simulink model "md11fl"  (Simulink 7.5)
settings: Solver=ode45  StartTime=0.0  StopTime=20  RelTol=1e-3
values from neighbouring files (symbols this model uses):
  alpha1f = 2.5e-7    (= 2.5e-07)    [gsnew2011.m]    (also in md11fla2011.m)
  alpha2f = 0.025    [gsnew2011.m]    (also in md11fla2011.m)
  alpha3f = 1    [gsnew2011.m]    (also in md11fla2011.m)
  ap = [Xu Xw 0 -g;Zu Zw Zq 0;Mu Mw Mq 0;0 0 1 0]    [gsnew2011.m]    (also in md11fla2011.m = [Xu Xw 0 -g 0;Zu Zw Zq 0 0;Mu Mw Mq 0 0;0 0 1 0 0;0 -1/U0  0)
  bp = [XL XT XR;ZL ZT ZR;ML MT MR;0 0 0]    [gsnew2011.m]    (also in md11fla2011.m = [XL XT XR;ZL ZT ZR;ML MT MR;0 0 0; 0 0 0])
  Cpf = [1 0 0 0 0 0 0 0;0 1 0 0 0 0 0 0;0 0 0 U0 0 0 0 0;0 0 0 0 1 0 0 0]    [md11fla2011.m]
  h_cr = 15    [gsnew2011.m]    (also in md11fla2011.m = 15000)
  Kfl1 = Kfl(:,1:8)    [md11fla2011.m]
  Kfl2 = Kgs(:,9:10)    [md11fla2011.m]
  ncon = 3    [gsnew2011.m]    (also in md11fla2011.m)
  np = 4    [gsnew2011.m]    (also in md11fla2011.m = 5)
  pthrot = 0.6    [gsnew2011.m]    (also in md11fla2011.m = 1)
  T2 = 200    [md11fla2011.m]
  tou = 1    [md11fla2011.m]
  u_ref = 0    [gsnew2011.m]    (also in md11fla2011.m = 165)
settings Model: Creator=ranjan  LastModifiedBy=knightofaccess
settings OptimizationCC: InitFltsAndDblsToZero=on
settings DebuggingCC: StrictBusMsg=Warning

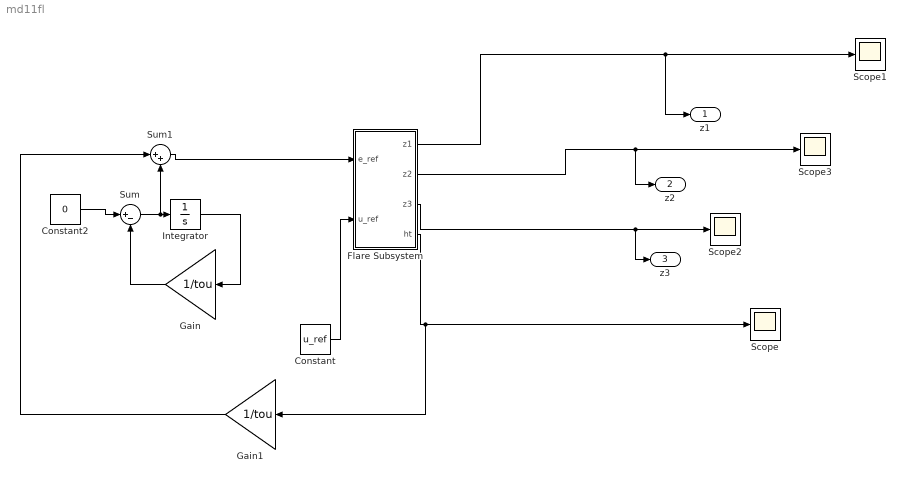
== system md11fl ==
  Constant : Constant  Value=u_ref  OutDataType=sfix(16)  OutScaling=2^0
  Constant2 : Constant  Value=0  OutDataType=sfix(16)  OutScaling=2^0
  Flare Subsystem : Subsystem
  Gain : Gain  Gain=1/tou  ParameterDataType=sfix(16)  ParameterScaling=2^0  OutDataType=sfix(16)  OutScaling=2^0
  Gain1 : Gain  Gain=1/tou  ParameterDataType=sfix(16)  ParameterScaling=2^0  OutDataType=sfix(16)  OutScaling=2^0
  Integrator : Integrator  InitialCondition=h_cr
  Scope{,1..3} (4 alike) : Scope
      Scope settings: YMin=-75600  YMax=-74950
      Scope2 settings: SaveName=ScopeData2
      Scope3 settings: SaveName=ScopeData3
  Sum : Sum  Inputs=|+-  OutDataType=sfix(16)  OutScaling=2^0
  Sum1 : Sum  Inputs=|++  OutDataType=sfix(16)  OutScaling=2^0
  z1 : Outport  OutDataType=sfix(16)  OutScaling=2^0
  z2 : Outport  Port=2  OutDataType=sfix(16)  OutScaling=2^0
  z3 : Outport  Port=3  OutDataType=sfix(16)  OutScaling=2^0
  wires:
  Constant/1 -> Flare Subsystem/2(u_ref)
  Flare Subsystem/1(z1) -> z1/1, Scope1/1
  Flare Subsystem/2(z2) -> z2/1, Scope3/1
  Flare Subsystem/3(z3) -> z3/1, Scope2/1
  Sum/1 -> Integrator/1, Sum1/2
  Constant2/1 -> Sum/1
  Integrator/1 -> Gain/1
  Gain/1 -> Sum/2
  Sum1/1 -> Flare Subsystem/1(e_ref)
  Flare Subsystem/4(ht) -> Scope/1, Gain1/1
  Gain1/1 -> Sum1/1

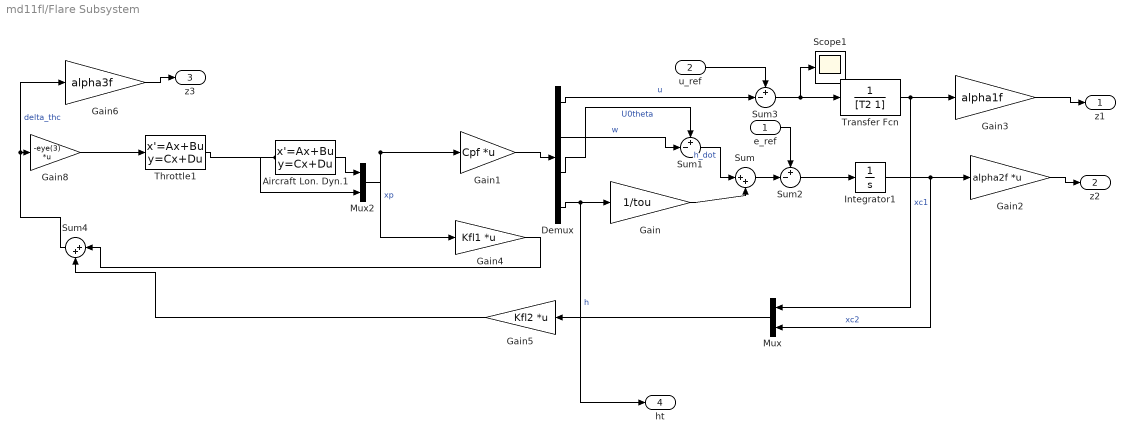
== system md11fl/Flare Subsystem ==
  e_ref : Inport  OutDataType=sfix(16)  OutScaling=2^0
  u_ref : Inport  Port=2  OutDataType=sfix(16)  OutScaling=2^0
  Aircraft Lon. Dyn.1 : StateSpace  A=ap  B=bp  C=eye(np)  D=zeros(np,3)
  Demux : Demux
  Gain : Gain  Gain=1/tou  ParameterDataType=sfix(16)  ParameterScaling=2^0  OutDataType=sfix(16)  OutScaling=2^0
  Gain1 : Gain  Gain=Cpf  Multiplication=Matrix(K*u)  ParameterDataType=sfix(16)  ParameterScaling=2^0  OutDataType=sfix(16)  OutScaling=2^0
  Gain2 : Gain  Gain=alpha2f  Multiplication=Matrix(K*u)  ParameterDataType=sfix(16)  ParameterScaling=2^0  OutDataType=sfix(16)  OutScaling=2^0
  Gain3 : Gain  Gain=alpha1f  ParameterDataType=sfix(16)  ParameterScaling=2^0  OutDataType=sfix(16)  OutScaling=2^0
  Gain4 : Gain  Gain=Kfl1  Multiplication=Matrix(K*u)  ParameterDataType=sfix(16)  ParameterScaling=2^0  OutDataType=sfix(16)  OutScaling=2^0
  Gain5 : Gain  Gain=Kfl2  Multiplication=Matrix(K*u)  ParameterDataType=sfix(16)  ParameterScaling=2^0  OutDataType=sfix(16)  OutScaling=2^0
  Gain6 : Gain  Gain=alpha3f  ParameterDataType=sfix(16)  ParameterScaling=2^0  OutDataType=sfix(16)  OutScaling=2^0
  Gain8 : Gain  Gain=-eye(3)  Multiplication=Matrix(K*u)  ParameterDataType=sfix(16)  ParameterScaling=2^0  OutDataType=sfix(16)  OutScaling=2^0
  Integrator1 : Integrator
  Mux : Mux  Inputs=2
  Mux2 : Mux  Inputs=2
  Scope1 : Scope
      settings: SaveName=ScopeData4
  Sum : Sum  Inputs=|++  OutDataType=sfix(16)  OutScaling=2^0
  Sum1 : Sum  Inputs=+-|  OutDataType=sfix(16)  OutScaling=2^0
  Sum2 : Sum  Inputs=+-|  OutDataType=sfix(16)  OutScaling=2^0
  Sum3 : Sum  Inputs=+-|  OutDataType=sfix(16)  OutScaling=2^0
  Sum4 : Sum  Inputs=|++  OutDataType=sfix(16)  OutScaling=2^0
  Throttle1 : StateSpace  A=-pthrot*eye(ncon)  B=pthrot*eye(ncon)  C=eye(3)  D=zeros(3,3)
  Transfer Fcn : TransferFcn  Denominator=[T2 1]
  z1 : Outport  OutDataType=sfix(16)  OutScaling=2^0
  z2 : Outport  Port=2  OutDataType=sfix(16)  OutScaling=2^0
  z3 : Outport  Port=3  OutDataType=sfix(16)  OutScaling=2^0
  ht : Outport  Port=4  OutDataType=sfix(16)  OutScaling=2^0
  wires:
  Mux2/1 -> Gain1/1, Gain4/1  "xp"
  Gain1/1 -> Demux/1
  Demux/2 -> Sum1/2  "w"
  Sum1/1 -> Sum/1  "h_dot"
  Gain/1 -> Sum/2
  Sum/1 -> Sum2/2
  e_ref/1 -> Sum2/1
  Sum2/1 -> Integrator1/1
  Demux/1 -> Sum3/2  "u"
  u_ref/1 -> Sum3/1
  Sum3/1 -> Transfer Fcn/1, Scope1/1
  Integrator1/1 -> Gain2/1, Mux/2  "xc2"
  Gain2/1 -> z2/1
  Transfer Fcn/1 -> Gain3/1, Mux/1  "xc1"
  Gain3/1 -> z1/1
  Mux/1 -> Gain5/1
  Gain5/1 -> Sum4/2
  Gain4/1 -> Sum4/1
  Sum4/1 -> Gain6/1, Gain8/1  "delta_thc"
  Gain6/1 -> z3/1
  Demux/4 -> Gain/1, ht/1  "h"
  Demux/3 -> Sum1/1  "U0theta"
  Aircraft Lon. Dyn.1/1 -> Mux2/1
  Throttle1/1 -> Aircraft Lon. Dyn.1/1, Mux2/2
  Gain8/1 -> Throttle1/1
